simulink model "mi_modelo_MI"  (R2022b)
settings: Solver=VariableStepAuto  StartTime=0.0  StopTime=250  RelTol=1e-3
undefined symbols (not defined in the file): DiscIntNeverNeededParam, fb, fd, J, kt, Lm, Lr, Ls, Rs, sg, Tr
libraries: neural x166
(part 4 of 5)

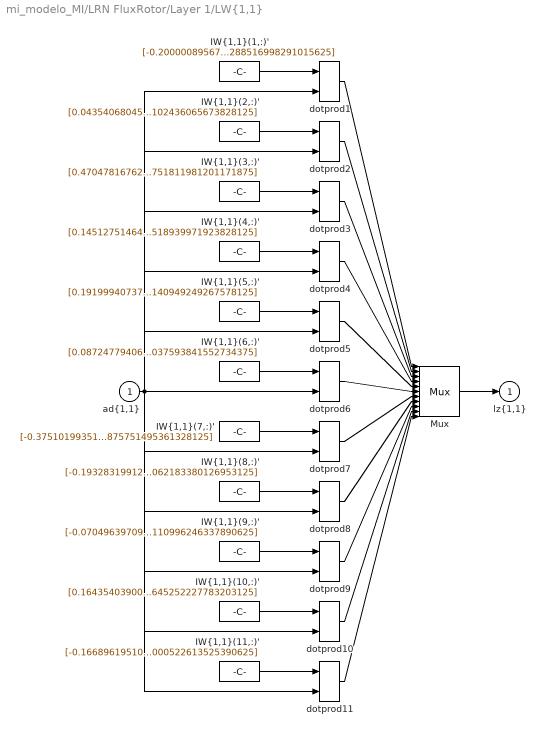
== system mi_modelo_MI/LRN FluxRotor/Layer 1/LW{1,1} ==
  "ad{1,1}" : Inport  PortDimensions=22  SampleTime=1
      mask Display: e = 0.06;c1 = [120 230 180]/255;c2 = ([120 230 180]+0)/(256+128);c3 = ([120 230 180]+128)/(256+128);patch([0 1 1 0],[0 0 1 1],c1);patch([0 1 1 1-e 1-e 0+e],[0 0 1 1-e 0+e 0+e],c2);patch([0 0 1 1-e 0+e 0+e],[0 1 1 1-e 1-e 0+e],c3);plot([0 1 1 0 0],[0 0 1 1 0]);
  "IW{1,1}(1,:)'" : Constant  Value=[-0.2000008956700982387655329830522532574832439422607421875;0.302996636376433314818967801329563371837139129638671875;0.1650278275068763900179646952892653644084930419921875;-0.408586841717532622819675225400715135037899017333984375;-0.04483203589571156666426787751333904452621936798095703125;0.035306798076872036862283721347921527922153472900390625;0.1875177470934279722047932636996847577393054962158203125;-0.056395436388283474993254884566340479068458080291748046875;-0.11263008689775690085443926591324270702898502349853515625;-0.0305415223256980360166945587252484983764588832855224609375;0.165920220492088821284681898760027252137660980224609375;-0.203273537191968223236671065023983828723430633544921875;0.317948071177563240663488386417157016694545745849609375;-0.052955797089628699192420668850900256074965000152587890625;-0.0576009386660631950149991098442114889621734619140625;0.1847234641577028824155348729618708603084087371826171875;0.03375325755650193659818114610970951616764068603515625;-0.0258204092253802065803913734498564735986292362213134765625;-0.1951232939831887558401746218805783428251743316650390625;-0.1803535264365876411574163284967653453350067138671875;0.043860703120889819872640913445138721726834774017333984375;0.060731147700970801450726099801613599993288516998291015625]
      mask Display: e = 0.06;c1 = [120 150 230]/255;c2 = ([120 150 230]+0)/383;c3 = ([120 150 230]+128)/383;patch([0 1 1 0],[0 0 1 1],c1);patch([0 1 1 1-e 1-e 0+e],[0 0 1 1-e 0+e 0+e],c2);patch([0 0 1 1-e 0+e 0+e],[0 1 1 1-e 1-e 0+e],c3);plot([0 1 1 0 0],[0 0 1 1 0]);disp('weights');
  "IW{1,1}(10,:)'" : Constant  Value=[0.16435403900055878256836194850620813667774200439453125;0.0289093186181135497481164975397405214607715606689453125;-0.0411189181845803275461292969339410774409770965576171875;-0.0686008595925789166347641412357916124165058135986328125;-0.0034032628003897876477201744904732549912296235561370849609375;-0.0792970652035882850316994563399930484592914581298828125;-0.10230610437406091606238334179579396732151508331298828125;-0.114362618871309662527124828557134605944156646728515625;0.11924062749464192645376670043333433568477630615234375;-0.05729452590242035958656430238988832570612430572509765625;-0.09464057802266818975045481465713237412273883819580078125;0.12450273869073787136318998136630398221313953399658203125;0.082886107215899063049846517969854176044464111328125;0.2217605719372452710569376677085529081523418426513671875;0.346469923394464307531137592377490364015102386474609375;0.2362943165241584153601905882169376127421855926513671875;0.06397660520491600666392884022570797242224216461181640625;-0.17262811934913269151792292177560739219188690185546875;-0.0117745681632965802643209229927379055880010128021240234375;-0.0080369246830075437293405826721937046386301517486572265625;0.162840064368928116866896971259848214685916900634765625;-0.0693962696305316928402362464112229645252227783203125]
      mask Display: e = 0.06;c1 = [120 150 230]/255;c2 = ([120 150 230]+0)/383;c3 = ([120 150 230]+128)/383;patch([0 1 1 0],[0 0 1 1],c1);patch([0 1 1 1-e 1-e 0+e],[0 0 1 1-e 0+e 0+e],c2);patch([0 0 1 1-e 0+e 0+e],[0 1 1 1-e 1-e 0+e],c3);plot([0 1 1 0 0],[0 0 1 1 0]);disp('weights');
  "IW{1,1}(11,:)'" : Constant  Value=[-0.1668961951074213467816065303850336931645870208740234375;0.08388531557141538919086798387070302851498126983642578125;-0.20064795718228811693961688433773815631866455078125;0.1708860408609948200453487743288860656321048736572265625;0.07091284575400232104147590916909393854439258575439453125;-0.3340017654954949843926215180545113980770111083984375;-0.077416802712458820945329307505744509398937225341796875;0.1343887781541462100864947615264100022614002227783203125;0.20373837125350824361902368764276616275310516357421875;0.01727727892918227980967316170790581963956356048583984375;0.06099128945166694404367291326707345433533191680908203125;-0.00660195090975303211511260315091931261122226715087890625;0.187460763751564118972936512363958172500133514404296875;-0.2281863995156795110741398957543424330651760101318359375;0.0719662211182572064682716472816537134349346160888671875;0.318292951081729669216002776011009700596332550048828125;-0.09514839379572477551239018112028134055435657501220703125;0.159963121792582096958312831702642142772674560546875;0.020243083576022037617381243990166694857180118560791015625;0.09553852678461882685923001190531067550182342529296875;-0.0031263420140322322436643442955528371385298669338226318359375;0.258268177768856299625355177340679802000522613525390625]
      mask Display: e = 0.06;c1 = [120 150 230]/255;c2 = ([120 150 230]+0)/383;c3 = ([120 150 230]+128)/383;patch([0 1 1 0],[0 0 1 1],c1);patch([0 1 1 1-e 1-e 0+e],[0 0 1 1-e 0+e 0+e],c2);patch([0 0 1 1-e 0+e 0+e],[0 1 1 1-e 1-e 0+e],c3);plot([0 1 1 0 0],[0 0 1 1 0]);disp('weights');
  "IW{1,1}(2,:)'" : Constant  Value=[0.043540680453497897228753998888350906781852245330810546875;-0.13467997995945280020890777450404129922389984130859375;-0.1380667927638561665037997272520442493259906768798828125;-0.2387783213449135022443670095526613295078277587890625;0.2310476160695549285861716271028853952884674072265625;-0.0859076366689631998330156648080446757376194000244140625;0.0877398939216627316017849125273642130196094512939453125;0.271221676775867226449889813011395744979381561279296875;-0.27224253081187199665436082796077243983745574951171875;0.29050932211973223839862612294382415711879730224609375;0.01361929517721961746534731219071545638144016265869140625;0.16703480574053075624618713845848105847835540771484375;0.33016889313436881270291678447392769157886505126953125;-0.435208308042706881746397584720398299396038055419921875;-0.1855758792702966453180835060265962965786457061767578125;0.1683756656842472498869511809971299953758716583251953125;0.007746014089674314699596191502450892585329711437225341796875;-0.08249085606413979199214026039044256322085857391357421875;-0.419452734537669458259045995873748324811458587646484375;-0.0970273495416597853147067098689149133861064910888671875;0.415305046198735094975518222781829535961151123046875;-0.037945943355370659322289839110453613102436065673828125]
      mask Display: e = 0.06;c1 = [120 150 230]/255;c2 = ([120 150 230]+0)/383;c3 = ([120 150 230]+128)/383;patch([0 1 1 0],[0 0 1 1],c1);patch([0 1 1 1-e 1-e 0+e],[0 0 1 1-e 0+e 0+e],c2);patch([0 0 1 1-e 0+e 0+e],[0 1 1 1-e 1-e 0+e],c3);plot([0 1 1 0 0],[0 0 1 1 0]);disp('weights');
  "IW{1,1}(3,:)'" : Constant  Value=[0.4704781676292040248910097943735308945178985595703125;0.1966818020255212129399069453938864171504974365234375;-0.042617587220815635051796022025882848538458347320556640625;0.246862714590145138071619612674112431704998016357421875;-0.2193320096527291707122486741354805417358875274658203125;0.02480000713369172327116274345826241187751293182373046875;0.355669714638014833330004194067441858351230621337890625;0.1302733275362366327509988650490413419902324676513671875;0.076811973185345994163952809685724787414073944091796875;0.1717346727873597933555771533065126277506351470947265625;-0.2037135372350467321655997920970548875629901885986328125;0.19148561404689512510657323218765668570995330810546875;0.276279263459079327258649527720990590751171112060546875;0.2270655441783554773227393752677016891539096832275390625;0.461643139318968886986027655439102090895175933837890625;-0.0217511096857220774525298878643297939561307430267333984375;0.006907591269496735943145271363619031035341322422027587890625;0.58238605804848886382529826732934452593326568603515625;0.2329070973159688140441403447766788303852081298828125;0.042435094958652219698791441260254941880702972412109375;0.37043995957129360885318192231352441012859344482421875;-0.156260499086052717654382604450802318751811981201171875]
      mask Display: e = 0.06;c1 = [120 150 230]/255;c2 = ([120 150 230]+0)/383;c3 = ([120 150 230]+128)/383;patch([0 1 1 0],[0 0 1 1],c1);patch([0 1 1 1-e 1-e 0+e],[0 0 1 1-e 0+e 0+e],c2);patch([0 0 1 1-e 0+e 0+e],[0 1 1 1-e 1-e 0+e],c3);plot([0 1 1 0 0],[0 0 1 1 0]);disp('weights');
  "IW{1,1}(4,:)'" : Constant  Value=[0.1451275146445129282657404701240011490881443023681640625;0.312916499419204463539045946163241751492023468017578125;0.58627677328621796704055668669752776622772216796875;-0.04071595547152608018937058886876911856234073638916015625;-0.199130943613760436061710379362921230494976043701171875;-0.22215806499735479828672168878256343305110931396484375;-0.06729153299937769283634025896390085108578205108642578125;0.22343444770519294007016242176177911460399627685546875;-0.01546345170250833234160126039569149725139141082763671875;-0.1653942326705824250598908520260010845959186553955078125;-0.30555610460089510649339672454516403377056121826171875;0.08776370058688807984648150295470259152352809906005859375;-0.05164280139901421262660363709073862992227077484130859375;-0.12314426159036249985856414923546253703534603118896484375;0.251952022417852139479776951702660880982875823974609375;-0.1529495584232792582124460523118614219129085540771484375;-0.1456348050647459368978076099665486253798007965087890625;-0.015000633636197226172814822575674043036997318267822265625;-0.0248960725614740148448067458275545504875481128692626953125;-0.11207587383229052069300024641052004881203174591064453125;-0.04214016978293384785292374772325274534523487091064453125;-0.259537924446202439288100549674709327518939971923828125]
      mask Display: e = 0.06;c1 = [120 150 230]/255;c2 = ([120 150 230]+0)/383;c3 = ([120 150 230]+128)/383;patch([0 1 1 0],[0 0 1 1],c1);patch([0 1 1 1-e 1-e 0+e],[0 0 1 1-e 0+e 0+e],c2);patch([0 0 1 1-e 0+e 0+e],[0 1 1 1-e 1-e 0+e],c3);plot([0 1 1 0 0],[0 0 1 1 0]);disp('weights');
  "IW{1,1}(5,:)'" : Constant  Value=[0.191999407374772002032869977483642287552356719970703125;0.225840180108502541767023785723722539842128753662109375;0.10215045947788735369865520397070213221013545989990234375;0.1766835604551550698015915941141429357230663299560546875;-0.0953223420962267808942414148987154476344585418701171875;-0.0696512777475846445174312293602270074188709259033203125;-0.17734597740302771029519135481677949428558349609375;0.1698788099504790205518389711869531311094760894775390625;-0.131357709517295251355761820377665571868419647216796875;-0.065518098927557222310724682756699621677398681640625;0.1474209529785487082786943346945918165147304534912109375;0.21197339751954535902456200346932746469974517822265625;0.215504514728298179893073438506689853966236114501953125;-0.0559440350424991461597556963170063681900501251220703125;0.068420594859693151246204934068373404443264007568359375;-0.11963100081169382449264304568714578635990619659423828125;-0.08005480701547547373042590379554894752800464630126953125;-0.2120411734117315927239388884117943234741687774658203125;-0.041290391272273095635281237036906532011926174163818359375;0.316369549722647358525051686228835023939609527587890625;0.042458513805174076527482185383632895536720752716064453125;-0.0285060977349291429228106409254905884154140949249267578125]
      mask Display: e = 0.06;c1 = [120 150 230]/255;c2 = ([120 150 230]+0)/383;c3 = ([120 150 230]+128)/383;patch([0 1 1 0],[0 0 1 1],c1);patch([0 1 1 1-e 1-e 0+e],[0 0 1 1-e 0+e 0+e],c2);patch([0 0 1 1-e 0+e 0+e],[0 1 1 1-e 1-e 0+e],c3);plot([0 1 1 0 0],[0 0 1 1 0]);disp('weights');
  "IW{1,1}(6,:)'" : Constant  Value=[0.08724779406578890561529959768449771218001842498779296875;-0.2562069844107421889844999896013177931308746337890625;0.2427080709301157879220767199512920342385768890380859375;-0.215359426162730793752331237556063570082187652587890625;-0.190367574444286924428837437517358921468257904052734375;0.224817621750374951883344465386471711099147796630859375;0.04554825918556042185780796671679127030074596405029296875;0.13906006854110819492831296884105540812015533447265625;-0.2287321073098151080760231934618786908686161041259765625;0.244129048260293635141948698219493962824344635009765625;-0.1742298276867547957014181747581460513174533843994140625;0.1555530583769197949806084579904563724994659423828125;0.0471989324613420191401047532053780741989612579345703125;0.1924375997100018498286999601987190544605255126953125;-0.03684191664960963230601720397316967137157917022705078125;-0.1324769954507019065204076468944549560546875;0.2538765627301824423511789063923060894012451171875;0.032581294119083857585561503356075263582170009613037109375;-0.1385753835042457249304703736925148405134677886962890625;-0.461876950637429339874273637178703211247920989990234375;0.3392840938329382272087286764872260391712188720703125;0.09554724490273534820428125158287002705037593841552734375]
      mask Display: e = 0.06;c1 = [120 150 230]/255;c2 = ([120 150 230]+0)/383;c3 = ([120 150 230]+128)/383;patch([0 1 1 0],[0 0 1 1],c1);patch([0 1 1 1-e 1-e 0+e],[0 0 1 1-e 0+e 0+e],c2);patch([0 0 1 1-e 0+e 0+e],[0 1 1 1-e 1-e 0+e],c3);plot([0 1 1 0 0],[0 0 1 1 0]);disp('weights');
  "IW{1,1}(7,:)'" : Constant  Value=[-0.3751019935141910455200786600471474230289459228515625;0.06080251323246148309475955784364487044513225555419921875;-0.1975914351124923584723802605367382057011127471923828125;0.0040891999961813300934476700376762892119586467742919921875;-0.2129068682527710809626597665555891580879688262939453125;-0.052912226277734154822329770695432671345770359039306640625;0.2035612598786275817541735477789188735187053680419921875;-0.07571071837164521090013380444361246190965175628662109375;0.116895578079847128893931085258373059332370758056640625;0.1267227425949099817170662163334782235324382781982421875;-0.10178086402175896829636059237600420601665973663330078125;-0.313842748691178397013601397702586837112903594970703125;-0.007198342679355248206751749506793203181587159633636474609375;0.100958155142178263030672269451315514743328094482421875;-0.00588723528709875730535738824755753739736974239349365234375;-0.158012875372274985696918747635209001600742340087890625;0.044961384700203825548481262330824392847716808319091796875;0.1964590986160929808601594004358048550784587860107421875;0.09545480007982047598869002058563637547194957733154296875;0.06939806152761462954003945924341678619384765625;0.041602191736428421886540007790244999341666698455810546875;0.1145407917939338660051618035140563733875751495361328125]
      mask Display: e = 0.06;c1 = [120 150 230]/255;c2 = ([120 150 230]+0)/383;c3 = ([120 150 230]+128)/383;patch([0 1 1 0],[0 0 1 1],c1);patch([0 1 1 1-e 1-e 0+e],[0 0 1 1-e 0+e 0+e],c2);patch([0 0 1 1-e 0+e 0+e],[0 1 1 1-e 1-e 0+e],c3);plot([0 1 1 0 0],[0 0 1 1 0]);disp('weights');
  "IW{1,1}(8,:)'" : Constant  Value=[-0.1932831991227903223329320780976559035480022430419921875;-0.58732162136867505086712526463088579475879669189453125;0.051064660990043274357841340815866715274751186370849609375;-0.077741022334313847341746850361232645809650421142578125;-0.05299442635062401318890579204889945685863494873046875;-0.011889956938229702398945875074787181802093982696533203125;-0.08875252860026215662170301357036805711686611175537109375;0.10356930443280644438264204154620529152452945709228515625;0.255178190608003896411304367575212381780147552490234375;-0.10764533772003141709472373577227699570357799530029296875;-0.0781746028442999729701767819278757087886333465576171875;-0.08968020943800673883128382612994755618274211883544921875;-0.233167566450394214694341599170002155005931854248046875;0.05546513490510375510300633550286875106394290924072265625;-0.06692474106079633611177115426471573300659656524658203125;-0.2584015465993474425232534485985524952411651611328125;-0.0001908556627702056619766413092520451755262911319732666015625;0.08192984626183234808660671433244715444743633270263671875;0.1790334590639393042010851786471903324127197265625;-0.048166718989651642612859205883069080300629138946533203125;-0.10313179216518804370839035300377872772514820098876953125;-0.186222019124293869385411426264909096062183380126953125]
      mask Display: e = 0.06;c1 = [120 150 230]/255;c2 = ([120 150 230]+0)/383;c3 = ([120 150 230]+128)/383;patch([0 1 1 0],[0 0 1 1],c1);patch([0 1 1 1-e 1-e 0+e],[0 0 1 1-e 0+e 0+e],c2);patch([0 0 1 1-e 0+e 0+e],[0 1 1 1-e 1-e 0+e],c3);plot([0 1 1 0 0],[0 0 1 1 0]);disp('weights');
  "IW{1,1}(9,:)'" : Constant  Value=[-0.070496397099968077792908616174827329814434051513671875;-0.048627362146768181305755973653504042886197566986083984375;-0.297798575094013973085793622885830700397491455078125;0.29028715165310503554252363755949772894382476806640625;0.0032884976270840496521963292053669647430069744586944580078125;-0.16958738780204585250288573661237023770809173583984375;0.0290589541272724682929862183300429023802280426025390625;-0.542302694534012363902775177848525345325469970703125;-0.0517459206814833427845456981231109239161014556884765625;0.257898404090294575130570819965214468538761138916015625;0.2337584983090739421118797736198757775127887725830078125;-0.0510049788836789141921457257922156713902950286865234375;-0.260631133850217466818577349840779788792133331298828125;0.26429675471970026645607276805094443261623382568359375;-0.131032064983700402560629072468145750463008880615234375;0.0024158347667139479231224186150939203798770904541015625;-0.0186409774822430020224661717520575621165335178375244140625;0.25169083218342225283237212352105416357517242431640625;-0.338143357357977791810554890616913326084613800048828125;0.2376779101393147464182931116738473065197467803955078125;0.30388577631497992737052982192835770547389984130859375;0.141122508840385629813596324311220087110996246337890625]
      mask Display: e = 0.06;c1 = [120 150 230]/255;c2 = ([120 150 230]+0)/383;c3 = ([120 150 230]+128)/383;patch([0 1 1 0],[0 0 1 1],c1);patch([0 1 1 1-e 1-e 0+e],[0 0 1 1-e 0+e 0+e],c2);patch([0 0 1 1-e 0+e 0+e],[0 1 1 1-e 1-e 0+e],c3);plot([0 1 1 0 0],[0 0 1 1 0]);disp('weights');
  Mux : Mux  Inputs=11
      mask Display: e = 0.06;c1 = [120 150 230]/255;c2 = ([120 150 230]+0)/383;c3 = ([120 150 230]+128)/383;patch([0 1 1 0],[0 0 1 1],c1);patch([0 1 1 1-e 1-e 0+e],[0 0 1 1-e 0+e 0+e],c2);patch([0 0 1 1-e 0+e 0+e],[0 1 1 1-e 1-e 0+e],c3);plot([0 1 1 0 0],[0 0 1 1 0]);disp('Mux');
  dotprod{1..11} (11 alike) : neural/Weight Functions/dotprod
  "lz{1,1}" : Outport
      mask Display: e = 0.06;c1 = [120 230 180]/255;c2 = ([120 230 180]+0)/(256+128);c3 = ([120 230 180]+128)/(256+128);patch([0 1 1 0],[0 0 1 1],c1);patch([0 1 1 1-e 1-e 0+e],[0 0 1 1-e 0+e 0+e],c2);patch([0 0 1 1-e 0+e 0+e],[0 1 1 1-e 1-e 0+e],c3);plot([0 1 1 0 0],[0 0 1 1 0]);
  wires:
  "IW{1,1}(1,:)'"/1 -> dotprod1/1
  "ad{1,1}"/1 -> dotprod1/2, dotprod2/2, dotprod3/2, dotprod4/2, dotprod5/2, dotprod6/2, dotprod7/2, dotprod8/2, dotprod9/2, dotprod10/2, dotprod11/2
  dotprod1/1 -> Mux/1
  "IW{1,1}(2,:)'"/1 -> dotprod2/1
  dotprod2/1 -> Mux/2
  "IW{1,1}(3,:)'"/1 -> dotprod3/1
  dotprod3/1 -> Mux/3
  "IW{1,1}(4,:)'"/1 -> dotprod4/1
  dotprod4/1 -> Mux/4
  "IW{1,1}(5,:)'"/1 -> dotprod5/1
  dotprod5/1 -> Mux/5
  "IW{1,1}(6,:)'"/1 -> dotprod6/1
  dotprod6/1 -> Mux/6
  "IW{1,1}(7,:)'"/1 -> dotprod7/1
  dotprod7/1 -> Mux/7
  "IW{1,1}(8,:)'"/1 -> dotprod8/1
  dotprod8/1 -> Mux/8
  "IW{1,1}(9,:)'"/1 -> dotprod9/1
  dotprod9/1 -> Mux/9
  "IW{1,1}(10,:)'"/1 -> dotprod10/1
  dotprod10/1 -> Mux/10
  "IW{1,1}(11,:)'"/1 -> dotprod11/1
  dotprod11/1 -> Mux/11
  Mux/1 -> "lz{1,1}"/1

== system mi_modelo_MI/LRN FluxRotor/Layer 2/Delays 1 ==
  "p{2}" : Inport  PortDimensions=11  SampleTime=1
      mask Display: e = 0.06;c1 = [120 230 180]/255;c2 = ([120 230 180]+0)/(256+128);c3 = ([120 230 180]+128)/(256+128);patch([0 1 1 0],[0 0 1 1],c1);patch([0 1 1 1-e 1-e 0+e],[0 0 1 1-e 0+e 0+e],c2);patch([0 0 1 1-e 0+e 0+e],[0 1 1 1-e 1-e 0+e],c3);plot([0 1 1 0 0],[0 0 1 1 0]);
  mux : Mux  Inputs=1
      mask Display: e = 0.06;c1 = [120 150 230]/255;c2 = ([120 150 230]+0)/383;c3 = ([120 150 230]+128)/383;patch([0 1 1 0],[0 0 1 1],c1);patch([0 1 1 1-e 1-e 0+e],[0 0 1 1-e 0+e 0+e],c2);patch([0 0 1 1-e 0+e 0+e],[0 1 1 1-e 1-e 0+e],c3);plot([0 1 1 0 0],[0 0 1 1 0]);disp('Mux')
  "pd{2,1}" : Outport
      mask Display: e = 0.06;c1 = [120 230 180]/255;c2 = ([120 230 180]+0)/(256+128);c3 = ([120 230 180]+128)/(256+128);patch([0 1 1 0],[0 0 1 1],c1);patch([0 1 1 1-e 1-e 0+e],[0 0 1 1-e 0+e 0+e],c2);patch([0 0 1 1-e 0+e 0+e],[0 1 1 1-e 1-e 0+e],c3);plot([0 1 1 0 0],[0 0 1 1 0]);
  wires:
  "p{2}"/1 -> mux/1
  mux/1 -> "pd{2,1}"/1

== system mi_modelo_MI/LRN FluxRotor/Layer 2/LW{2,1} ==
  "ad{2,1}" : Inport  PortDimensions=11  SampleTime=1
      mask Display: e = 0.06;c1 = [120 230 180]/255;c2 = ([120 230 180]+0)/(256+128);c3 = ([120 230 180]+128)/(256+128);patch([0 1 1 0],[0 0 1 1],c1);patch([0 1 1 1-e 1-e 0+e],[0 0 1 1-e 0+e 0+e],c2);patch([0 0 1 1-e 0+e 0+e],[0 1 1 1-e 1-e 0+e],c3);plot([0 1 1 0 0],[0 0 1 1 0]);
  "IW{2,1}(1,:)'" : Constant  Value=[-0.06868717582190109194328897501691244542598724365234375;0.62472657970267331251079667708836495876312255859375;0.44503813316579587944232798690791241824626922607421875;-0.367716543932283757012413616394042037427425384521484375;0.049712296129675141720394293542995001189410686492919921875;-0.663788730614703670340759344981051981449127197265625;-0.56999601753901918410605276221758686006069183349609375;-0.279641082269581564556659714071429334580898284912109375;-0.7705190310706757639280795046943239867687225341796875;0.4197412101683555274433956583379767835140228271484375;-0.5568656180794226973063132390961982309818267822265625]
      mask Display: e = 0.06;c1 = [120 150 230]/255;c2 = ([120 150 230]+0)/383;c3 = ([120 150 230]+128)/383;patch([0 1 1 0],[0 0 1 1],c1);patch([0 1 1 1-e 1-e 0+e],[0 0 1 1-e 0+e 0+e],c2);patch([0 0 1 1-e 0+e 0+e],[0 1 1 1-e 1-e 0+e],c3);plot([0 1 1 0 0],[0 0 1 1 0]);disp('weights');
  "IW{2,1}(2,:)'" : Constant  Value=[-0.1852697121457130557953263405579491518437862396240234375;-0.45166136798426970155873050316586159169673919677734375;0.61088630781476538356145056241075508296489715576171875;0.598979443912593279009115576627664268016815185546875;0.6099032528007797271385470594395883381366729736328125;-0.179606056893742038749195444324868731200695037841796875;0.38838808430518112491114379736245609819889068603515625;-1.1269915629088813613378761147032491862773895263671875;0.377232396775045220049804584050434641540050506591796875;0.00788094970440296992142403809111783630214631557464599609375;-0.05715279658647028082629759637711686082184314727783203125]
      mask Display: e = 0.06;c1 = [120 150 230]/255;c2 = ([120 150 230]+0)/383;c3 = ([120 150 230]+128)/383;patch([0 1 1 0],[0 0 1 1],c1);patch([0 1 1 1-e 1-e 0+e],[0 0 1 1-e 0+e 0+e],c2);patch([0 0 1 1-e 0+e 0+e],[0 1 1 1-e 1-e 0+e],c3);plot([0 1 1 0 0],[0 0 1 1 0]);disp('weights');
  Mux : Mux  Inputs=2
      mask Display: e = 0.06;c1 = [120 150 230]/255;c2 = ([120 150 230]+0)/383;c3 = ([120 150 230]+128)/383;patch([0 1 1 0],[0 0 1 1],c1);patch([0 1 1 1-e 1-e 0+e],[0 0 1 1-e 0+e 0+e],c2);patch([0 0 1 1-e 0+e 0+e],[0 1 1 1-e 1-e 0+e],c3);plot([0 1 1 0 0],[0 0 1 1 0]);disp('Mux');
  dotprod1 : neural/Weight Functions/dotprod
  dotprod2 : neural/Weight Functions/dotprod
  "lz{2,1}" : Outport
      mask Display: e = 0.06;c1 = [120 230 180]/255;c2 = ([120 230 180]+0)/(256+128);c3 = ([120 230 180]+128)/(256+128);patch([0 1 1 0],[0 0 1 1],c1);patch([0 1 1 1-e 1-e 0+e],[0 0 1 1-e 0+e 0+e],c2);patch([0 0 1 1-e 0+e 0+e],[0 1 1 1-e 1-e 0+e],c3);plot([0 1 1 0 0],[0 0 1 1 0]);
  wires:
  "IW{2,1}(1,:)'"/1 -> dotprod1/1
  "ad{2,1}"/1 -> dotprod1/2, dotprod2/2
  dotprod1/1 -> Mux/1
  "IW{2,1}(2,:)'"/1 -> dotprod2/1
  dotprod2/1 -> Mux/2
  Mux/1 -> "lz{2,1}"/1

== system mi_modelo_MI/NARX WR/Layer 1/Delays 1 ==
  "p{1}" : Inport  PortDimensions=4  SampleTime=1
      mask Display: e = 0.06;c1 = [120 230 180]/255;c2 = ([120 230 180]+0)/(256+128);c3 = ([120 230 180]+128)/(256+128);patch([0 1 1 0],[0 0 1 1],c1);patch([0 1 1 1-e 1-e 0+e],[0 0 1 1-e 0+e 0+e],c2);patch([0 0 1 1-e 0+e 0+e],[0 1 1 1-e 1-e 0+e],c3);plot([0 1 1 0 0],[0 0 1 1 0]);
  Delay 1 : UnitDelay  InitialCondition=pi_input_1_delayed_1
      mask Display: e = 0.06;c1 = [120 150 230]/255;c2 = ([120 150 230]+0)/383;c3 = ([120 150 230]+128)/383;patch([0 1 1 0],[0 0 1 1],c1);patch([0 1 1 1-e 1-e 0+e],[0 0 1 1-e 0+e 0+e],c2);patch([0 0 1 1-e 0+e 0+e],[0 1 1 1-e 1-e 0+e],c3);plot([0 1 1 0 0],[0 0 1 1 0]);disp('D')
  Delay 2 : UnitDelay  InitialCondition=pi_input_1_delayed_2
      mask Display: e = 0.06;c1 = [120 150 230]/255;c2 = ([120 150 230]+0)/383;c3 = ([120 150 230]+128)/383;patch([0 1 1 0],[0 0 1 1],c1);patch([0 1 1 1-e 1-e 0+e],[0 0 1 1-e 0+e 0+e],c2);patch([0 0 1 1-e 0+e 0+e],[0 1 1 1-e 1-e 0+e],c3);plot([0 1 1 0 0],[0 0 1 1 0]);disp('D')
  mux : Mux  Inputs=2
      mask Display: e = 0.06;c1 = [120 150 230]/255;c2 = ([120 150 230]+0)/383;c3 = ([120 150 230]+128)/383;patch([0 1 1 0],[0 0 1 1],c1);patch([0 1 1 1-e 1-e 0+e],[0 0 1 1-e 0+e 0+e],c2);patch([0 0 1 1-e 0+e 0+e],[0 1 1 1-e 1-e 0+e],c3);plot([0 1 1 0 0],[0 0 1 1 0]);disp('Mux')
  "pd{1,1}" : Outport
      mask Display: e = 0.06;c1 = [120 230 180]/255;c2 = ([120 230 180]+0)/(256+128);c3 = ([120 230 180]+128)/(256+128);patch([0 1 1 0],[0 0 1 1],c1);patch([0 1 1 1-e 1-e 0+e],[0 0 1 1-e 0+e 0+e],c2);patch([0 0 1 1-e 0+e 0+e],[0 1 1 1-e 1-e 0+e],c3);plot([0 1 1 0 0],[0 0 1 1 0]);
  wires:
  "p{1}"/1 -> Delay 1/1
  Delay 1/1 -> Delay 2/1, mux/1
  Delay 2/1 -> mux/2
  mux/1 -> "pd{1,1}"/1

== system mi_modelo_MI/NARX WR/Layer 1/Delays 2 ==
  "p{1}" : Inport  PortDimensions=1  SampleTime=1
      mask Display: e = 0.06;c1 = [120 230 180]/255;c2 = ([120 230 180]+0)/(256+128);c3 = ([120 230 180]+128)/(256+128);patch([0 1 1 0],[0 0 1 1],c1);patch([0 1 1 1-e 1-e 0+e],[0 0 1 1-e 0+e 0+e],c2);patch([0 0 1 1-e 0+e 0+e],[0 1 1 1-e 1-e 0+e],c3);plot([0 1 1 0 0],[0 0 1 1 0]);
  Delay 1 : UnitDelay  InitialCondition=ai_layer_2_delayed_1
      mask Display: e = 0.06;c1 = [120 150 230]/255;c2 = ([120 150 230]+0)/383;c3 = ([120 150 230]+128)/383;patch([0 1 1 0],[0 0 1 1],c1);patch([0 1 1 1-e 1-e 0+e],[0 0 1 1-e 0+e 0+e],c2);patch([0 0 1 1-e 0+e 0+e],[0 1 1 1-e 1-e 0+e],c3);plot([0 1 1 0 0],[0 0 1 1 0]);disp('D')
  Delay 2 : UnitDelay  InitialCondition=ai_layer_2_delayed_2
      mask Display: e = 0.06;c1 = [120 150 230]/255;c2 = ([120 150 230]+0)/383;c3 = ([120 150 230]+128)/383;patch([0 1 1 0],[0 0 1 1],c1);patch([0 1 1 1-e 1-e 0+e],[0 0 1 1-e 0+e 0+e],c2);patch([0 0 1 1-e 0+e 0+e],[0 1 1 1-e 1-e 0+e],c3);plot([0 1 1 0 0],[0 0 1 1 0]);disp('D')
  mux : Mux  Inputs=2
      mask Display: e = 0.06;c1 = [120 150 230]/255;c2 = ([120 150 230]+0)/383;c3 = ([120 150 230]+128)/383;patch([0 1 1 0],[0 0 1 1],c1);patch([0 1 1 1-e 1-e 0+e],[0 0 1 1-e 0+e 0+e],c2);patch([0 0 1 1-e 0+e 0+e],[0 1 1 1-e 1-e 0+e],c3);plot([0 1 1 0 0],[0 0 1 1 0]);disp('Mux')
  "pd{1,2}" : Outport
      mask Display: e = 0.06;c1 = [120 230 180]/255;c2 = ([120 230 180]+0)/(256+128);c3 = ([120 230 180]+128)/(256+128);patch([0 1 1 0],[0 0 1 1],c1);patch([0 1 1 1-e 1-e 0+e],[0 0 1 1-e 0+e 0+e],c2);patch([0 0 1 1-e 0+e 0+e],[0 1 1 1-e 1-e 0+e],c3);plot([0 1 1 0 0],[0 0 1 1 0]);
  wires:
  "p{1}"/1 -> Delay 1/1
  Delay 1/1 -> Delay 2/1, mux/1
  Delay 2/1 -> mux/2
  mux/1 -> "pd{1,2}"/1
